simulink model "Image_Processing_Test"  (R2024b)
settings: Solver=VariableStepAuto  StartTime=0.0  StopTime=100  RelTol=1e-3
undefined symbols (not defined in the file or in its folder): RGB
libraries: zeromq_image_lib x9
settings Model: Creator=tkami  LastModifiedBy=tkami

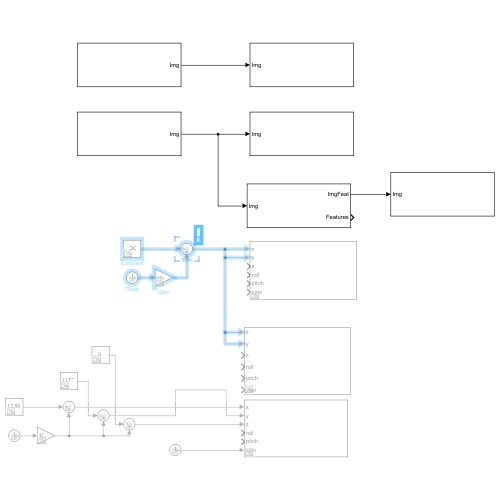
[thumbnail: Simulink's stored preview of the top-level diagram]
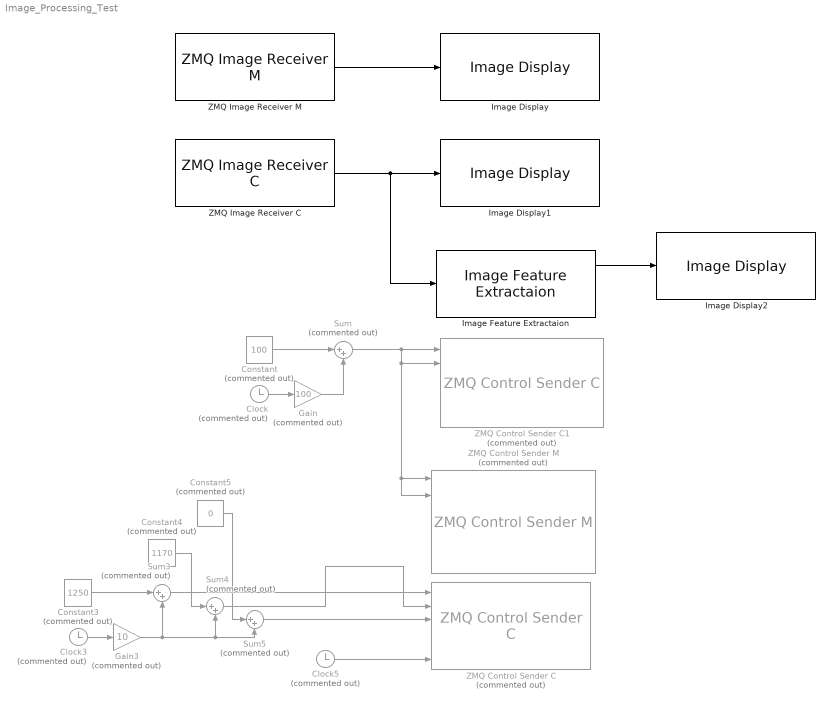
== system Image_Processing_Test ==
  Clock : Clock  Commented=on
  Clock3 : Clock  Commented=on
  Clock5 : Clock  Commented=on
  Constant : Constant  Commented=on  Value=100
  Constant3 : Constant  Commented=on  Value=1250
  Constant4 : Constant  Commented=on  Value=1170
  Constant5 : Constant  Commented=on  Value=0
  Gain : Gain  Commented=on  Gain=100
  Gain3 : Gain  Commented=on  Gain=10
  Image Display : zeromq_image_lib/Image Display  imgHeight=1024  imgWidth=1024  channels=3 (RGB)  title=ZeroMQ Image Display  decimation=1  sample_time=1
      settings: SourceProductName=ZeroMQ Image Processing
  Image Display1 : zeromq_image_lib/Image Display  imgHeight=1024  imgWidth=1024  channels=3 (RGB)  title=ZeroMQ Image Display  decimation=1  sample_time=1
      settings: SourceProductName=ZeroMQ Image Processing
  Image Display2 : zeromq_image_lib/Image Display  imgHeight=1024  imgWidth=1024  channels=3 (RGB)  title=ZeroMQ Image Display  decimation=1  sample_time=1
      settings: SourceProductName=ZeroMQ Image Processing
  Image Feature Extractaion : zeromq_image_lib/Image Feature Extractaion  imgHeight=1024  imgWidth=1024  channels=3  processingMode=ORB Features  nfeatures=500  threshold=127  sample_time=-1  enable_logging=on
      settings: SourceProductName=ZeroMQ Image Processing
  Sum{,3..5} (4 alike) : Sum  Commented=on  Inputs=|++
  ZMQ Control Sender C : zeromq_image_lib/ZMQ Control Sender C  Commented=on  address=tcp://127.0.0.1:5559  target_id_default=Actor01  sample_time=0.0625  enable_logging=off
      settings: SourceProductName=ZeroMQ Image Processing
  ZMQ Control Sender C1 : zeromq_image_lib/ZMQ Control Sender C  Commented=on  address=tcp://127.0.0.1:5556  target_id_default=Camera01  sample_time=0.0625  enable_logging=off
      settings: SourceProductName=ZeroMQ Image Processing
  ZMQ Control Sender M : zeromq_image_lib/ZMQ Control Sender M  Commented=on  address=tcp://127.0.0.1:5556  target_id_default=Camera01  sample_time=0.0625  enable_logging=off
      settings: SourceProductName=ZeroMQ Image Processing
  ZMQ Image Receiver C : zeromq_image_lib/ZMQ Image Receiver C  address=tcp://127.0.0.1:5555  camera_id=Camera01  bind_mode=off  timeout_ms=1000  imgHeight=1024  imgWidth=1024  channels=3 (RGB)  sample_time=1  enable_logging=off
      settings: SourceProductName=ZeroMQ Image Processing
  ZMQ Image Receiver M : zeromq_image_lib/ZMQ Image Receiver M  address=tcp://127.0.0.1:5555  camera_id=Camera01  bind_mode=off  timeout_ms=1000  imgHeight=1024  imgWidth=1024  channels=3 (RGB)  sample_time=1  enable_logging=off  save_debug_image=off
      settings: SourceProductName=ZeroMQ Image Processing
  wires:
  Constant/1 -> Sum/1
  Sum/1 -> ZMQ Control Sender C1/1, ZMQ Control Sender C1/2, ZMQ Control Sender M/2, ZMQ Control Sender M/1
  Clock/1 -> Gain/1
  Gain/1 -> Sum/2
  ZMQ Image Receiver M/1 -> Image Display/1
  Gain3/1 -> Sum5/2, Sum4/2, Sum3/2
  Clock3/1 -> Gain3/1
  Constant3/1 -> Sum3/1
  Constant4/1 -> Sum4/1
  Constant5/1 -> Sum5/1
  Sum3/1 -> ZMQ Control Sender C/1
  Sum4/1 -> ZMQ Control Sender C/2
  Sum5/1 -> ZMQ Control Sender C/3
  ZMQ Image Receiver C/1 -> Image Feature Extractaion/1, Image Display1/1
  Clock5/1 -> ZMQ Control Sender C/6
  Image Feature Extractaion/1 -> Image Display2/1
